simulink model "Blocks391"  (R2017a)
settings: Solver=VariableStepAuto  StartTime=0.0  StopTime=10.0  RelTol=1e-3
values from neighbouring files (symbols this model uses):
  motorxd = cell2mat(motorxd)    [System391.m]
  motorxn = cell2mat(motorxn)    [System391.m]
  motoryd = motorxd    [Control391.m]
  motoryn = motorxn    [Control391.m]
  PIDX = [KpX KiX KdX]    [Control391.m]
  PIDY = [KpY KiY KdY]    [Control391.m]
libraries: simulink x6
settings Model: Creator=seung  LastModifiedBy=seung

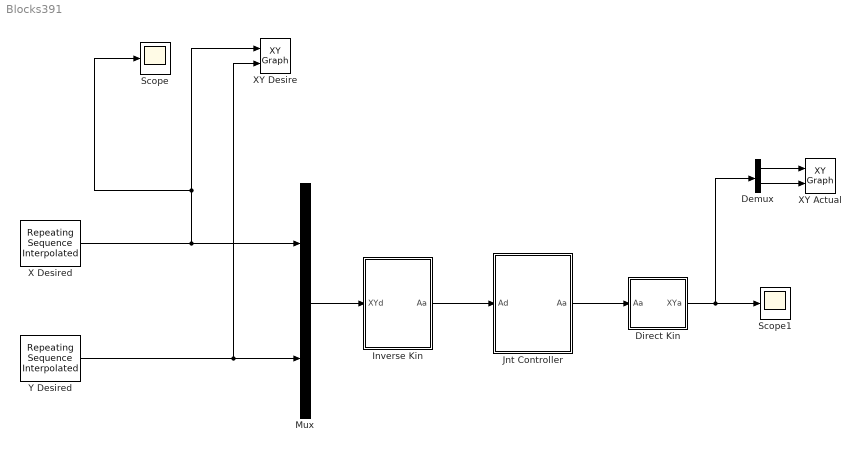
== system Blocks391 ==
  Demux : Demux  Outputs=2
  Direct Kin : Subsystem
  Inverse Kin : Subsystem
  Jnt Controller : Subsystem
  Mux : Mux  Inputs=2
  Scope : Scope
  Scope1 : Scope
  X Desired : simulink/Sources/Repeating Sequence Interpolated  OutValues=Xtest  TimeValues=Timetest  LookUpMeth=Interpolation-Use End Values  tsamp=SampleTimetest  OutMin=[]  OutMax=[]  OutDataTypeStr=double  OutputDataTypeScalingMode=double  OutDataType=fixdt(0,8)  OutScaling=2^-10
  XY Actual : simulink/Sinks/XY Graph  xmin=0  xmax=10  ymin=0  ymax=10  st=-1
  "XY Desire " : simulink/Sinks/XY Graph  xmin=0  xmax=10  ymin=0  ymax=10  st=-1
  Y Desired : simulink/Sources/Repeating Sequence Interpolated  OutValues=Ytest  TimeValues=Timetest  LookUpMeth=Interpolation-Use End Values  tsamp=SampleTimetest  OutMin=[]  OutMax=[]  OutDataTypeStr=double  OutputDataTypeScalingMode=double  OutDataType=fixdt(0,8)  OutScaling=2^-10
  wires:
  Y Desired/1 -> Mux/2, "XY Desire "/2
  X Desired/1 -> "XY Desire "/1, Scope/1, Mux/1
  Mux/1 -> Inverse Kin/1("XYd ")
  Inverse Kin/1(Aa) -> Jnt Controller/1("Ad ")
  Jnt Controller/1(Aa) -> Direct Kin/1(Aa)
  Direct Kin/1(XYa) -> Demux/1, Scope1/1
  Demux/2 -> XY Actual/2
  Demux/1 -> XY Actual/1

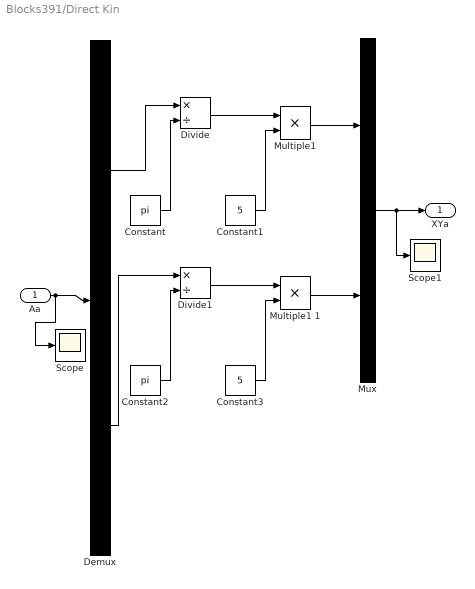
== system Blocks391/Direct Kin ==
  Aa : Inport
  Constant : Constant  Value=pi
  Constant1 : Constant  Value=5
  Constant2 : Constant  Value=pi
  Constant3 : Constant  Value=5
  Demux : Demux  Outputs=2
  Divide : Product  Inputs=*/
  Divide1 : Product  Inputs=*/
  "Multiple1 " : Product  Inputs=**
  Multiple1 1 : Product  Inputs=**
  Mux : Mux  Inputs=2
  Scope : Scope
  Scope1 : Scope
  XYa : Outport
  wires:
  Aa/1 -> Scope/1, Demux/1
  Mux/1 -> Scope1/1, XYa/1
  Divide/1 -> "Multiple1 "/1
  "Multiple1 "/1 -> Mux/1
  Demux/1 -> Divide/1
  Constant/1 -> Divide/2
  Constant1/1 -> "Multiple1 "/2
  Divide1/1 -> Multiple1 1/1
  Multiple1 1/1 -> Mux/2
  Constant3/1 -> Multiple1 1/2
  Constant2/1 -> Divide1/2
  Demux/2 -> Divide1/1

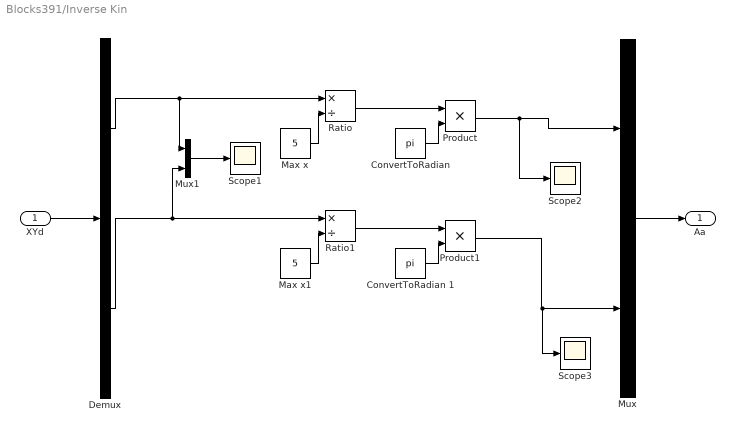
== system Blocks391/Inverse Kin ==
  "XYd " : Inport
  " ConvertToRadian " : Constant  Value=pi
  " ConvertToRadian 1" : Constant  Value=pi
  Demux : Demux  Outputs=2
  Max x : Constant  Value=5
  Max x1 : Constant  Value=5
  Mux : Mux  Inputs=2
  Mux1 : Mux  Inputs=2
  Product : Product
  Product1 : Product
  Ratio : Product  Inputs=*/
  Ratio1 : Product  Inputs=*/
  Scope1 : Scope
  Scope2 : Scope
  Scope3 : Scope
  Aa : Outport
  wires:
  "XYd "/1 -> Demux/1
  Mux/1 -> Aa/1
  Demux/1 -> Mux1/1, Ratio/1
  Demux/2 -> Mux1/2, Ratio1/1
  Ratio/1 -> Product/1
  Mux1/1 -> Scope1/1
  Max x/1 -> Ratio/2
  " ConvertToRadian "/1 -> Product/2
  Ratio1/1 -> Product1/1
  " ConvertToRadian 1"/1 -> Product1/2
  Max x1/1 -> Ratio1/2
  Product1/1 -> Scope3/1, Mux/2
  Product/1 -> Scope2/1, Mux/1

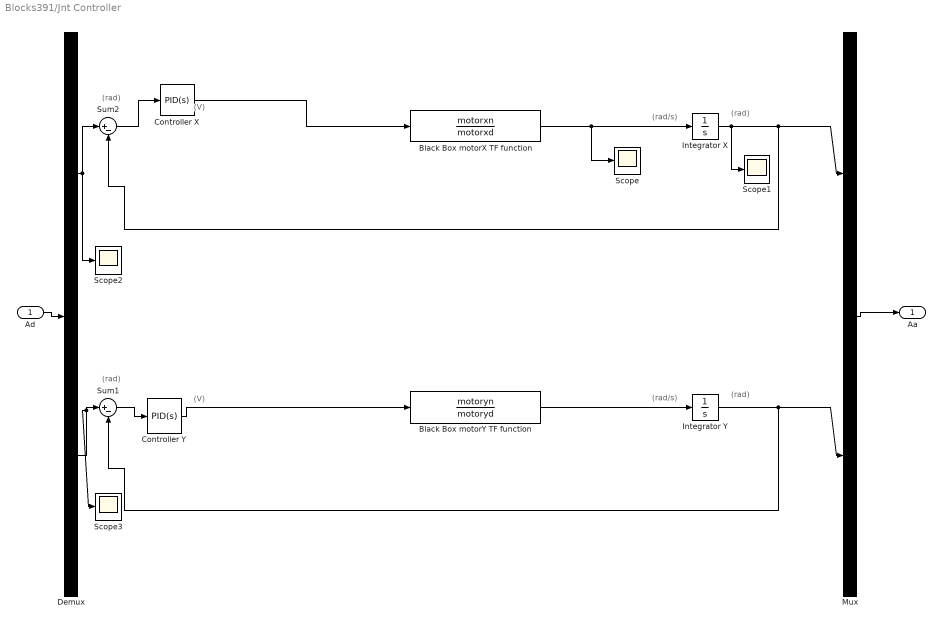
== system Blocks391/Jnt Controller ==
  note: (V)
  note: (rad/s)
  note: (rad)
  note: (rad)
  note: (V)
  note: (rad/s)
  note: (rad)
  note: (rad)
  "Ad " : Inport
  "Black Box motorX TF function " : TransferFcn  Numerator=motorxn  Denominator=motorxd
  "Black Box motorY TF function " : TransferFcn  Numerator=motoryn  Denominator=motoryd
  Controller X : simulink/Continuous/PID Controller  Controller=PID  TimeDomain=Continuous-time  SampleTime=-1  IntegratorMethod=Forward Euler  FilterMethod=Forward Euler  Form=Parallel  UseFilter=on  ControllerParametersSource=internal  P=PIDX(1)  I=PIDX(2)  D=PIDX(3)  N=100  InitialConditionSource=internal  InitialConditionForIntegrator=0  InitialConditionForFilter=0  ExternalReset=none  LimitOutput=off  UpperSaturationLimit=inf  LowerSaturationLimit=-inf  LinearizeAsGain=on  AntiWindupMode=none  Kb=1  TrackingMode=off  Kt=1  PParamMin=[]  PParamMax=[]  IParamMin=[]  IParamMax=[]  DParamMin=[]  DParamMax=[]  NParamMin=[]  NParamMax=[]  KbParamMin=[]  KbParamMax=[]  KtParamMin=[]  KtParamMax=[]  POutMin=[]  POutMax=[]  IOutMin=[]  IOutMax=[]  DOutMin=[]  DOutMax=[]  NOutMin=[]  NOutMax=[]  KbOutMin=[]  KbOutMax=[]  KtOutMin=[]  KtOutMax=[]  IntegratorOutMin=[]  IntegratorOutMax=[]  FilterOutMin=[]  FilterOutMax=[]  SumOutMin=[]  SumOutMax=[]  SumI1OutMin=[]  SumI1OutMax=[]  SumI2OutMin=[]  SumI2OutMax=[]  SumI3OutMin=[]  SumI3OutMax=[]  SumDOutMin=[]  SumDOutMax=[]  SaturationOutMin=[]  SaturationOutMax=[]  IntegratorContinuousStateAttributes=''  IntegratorStateMustResolveToSignalObject=off  IntegratorRTWStateStorageClass=Auto  FilterContinuousStateAttributes=''  FilterStateMustResolveToSignalObject=off  FilterRTWStateStorageClass=Auto  DifferentiatorICPrevScaledInput=0  DifferentiatorOutMin=[]  DifferentiatorOutMax=[]  InitialConditionSetting=State (most efficient)
  Controller Y : simulink/Continuous/PID Controller  Controller=PID  TimeDomain=Continuous-time  SampleTime=-1  IntegratorMethod=Forward Euler  FilterMethod=Forward Euler  Form=Parallel  UseFilter=on  ControllerParametersSource=internal  P=PIDY(1)  I=PIDY(2)  D=PIDY(3)  N=100  InitialConditionSource=internal  InitialConditionForIntegrator=0  InitialConditionForFilter=0  ExternalReset=none  LimitOutput=off  UpperSaturationLimit=inf  LowerSaturationLimit=-inf  LinearizeAsGain=on  AntiWindupMode=none  Kb=1  TrackingMode=off  Kt=1  PParamMin=[]  PParamMax=[]  IParamMin=[]  IParamMax=[]  DParamMin=[]  DParamMax=[]  NParamMin=[]  NParamMax=[]  KbParamMin=[]  KbParamMax=[]  KtParamMin=[]  KtParamMax=[]  POutMin=[]  POutMax=[]  IOutMin=[]  IOutMax=[]  DOutMin=[]  DOutMax=[]  NOutMin=[]  NOutMax=[]  KbOutMin=[]  KbOutMax=[]  KtOutMin=[]  KtOutMax=[]  IntegratorOutMin=[]  IntegratorOutMax=[]  FilterOutMin=[]  FilterOutMax=[]  SumOutMin=[]  SumOutMax=[]  SumI1OutMin=[]  SumI1OutMax=[]  SumI2OutMin=[]  SumI2OutMax=[]  SumI3OutMin=[]  SumI3OutMax=[]  SumDOutMin=[]  SumDOutMax=[]  SaturationOutMin=[]  SaturationOutMax=[]  IntegratorContinuousStateAttributes=''  IntegratorStateMustResolveToSignalObject=off  IntegratorRTWStateStorageClass=Auto  FilterContinuousStateAttributes=''  FilterStateMustResolveToSignalObject=off  FilterRTWStateStorageClass=Auto  DifferentiatorICPrevScaledInput=0  DifferentiatorOutMin=[]  DifferentiatorOutMax=[]  InitialConditionSetting=State (most efficient)
  Demux : Demux  Outputs=2
  Integrator X : Integrator
  Integrator Y : Integrator
  Mux : Mux  Inputs=2
  Scope{,1..3} (4 alike) : Scope
  Sum1 : Sum  Inputs=|+-
  Sum2 : Sum  Inputs=|+-
  Aa : Outport
  wires:
  "Ad "/1 -> Demux/1
  Mux/1 -> Aa/1
  Demux/1 -> Scope2/1, Sum2/1
  Integrator X/1 -> Scope1/1, Sum2/2, Mux/1
  "Black Box motorX TF function "/1 -> Scope/1, Integrator X/1
  Demux/2 -> Scope3/1, Sum1/1
  Integrator Y/1 -> Mux/2, Sum1/2
  "Black Box motorY TF function "/1 -> Integrator Y/1
  Sum2/1 -> Controller X/1
  Controller X/1 -> "Black Box motorX TF function "/1
  Sum1/1 -> Controller Y/1
  Controller Y/1 -> "Black Box motorY TF function "/1
